simulink model "Finalproject342"  (R2014b)
settings: Solver=ode113  StartTime=0.0  StopTime=1200  RelTol=1e-3
undefined symbols (not defined in the file): ln
settings Model: Creator=mdbell  LastModifiedBy=Mike
settings DebuggingCC: MaxConsecutiveZCsMsg=none

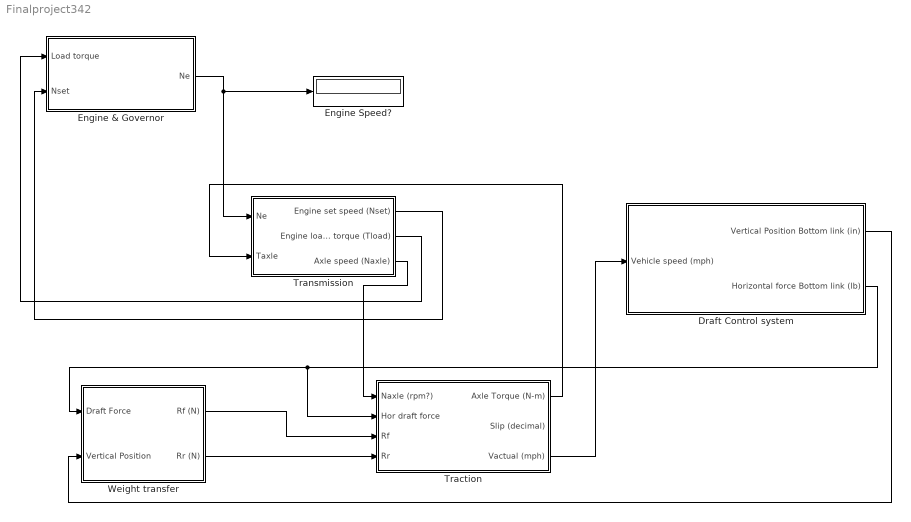
== system Finalproject342 ==
  Draft Control system : Subsystem
  Engine & Governor : Subsystem
  Engine Speed? : Display
  Traction : Subsystem
  Transmission : Subsystem
  Weight transfer : Subsystem
  wires:
  Engine & Governor/1(Ne) -> Transmission/1(Ne), Engine Speed?/1
  Transmission/1(Engine set speed (Nset)) -> Engine & Governor/2("Nset ")
  Draft Control system/2(Horizontal force Bottom link (lb)) -> Traction/2(Hor draft force), Weight transfer/1(Draft Force)
  Draft Control system/1(Vertical Position Bottom link (in)) -> Weight transfer/2(Vertical Position)
  Weight transfer/1(Rf (N)) -> Traction/3(Rf)
  Weight transfer/2(Rr (N)) -> Traction/4(Rr)
  Transmission/3(Axle speed (Naxle)) -> Traction/1(Naxle (rpm?))
  Traction/1(Axle Torque (N-m)) -> Transmission/2(Taxle)
  Traction/3(Vactual (mph)) -> Draft Control system/1(Vehicle speed (mph))
  Transmission/2(Engine load torque (Tload)) -> Engine & Governor/1(Load torque)

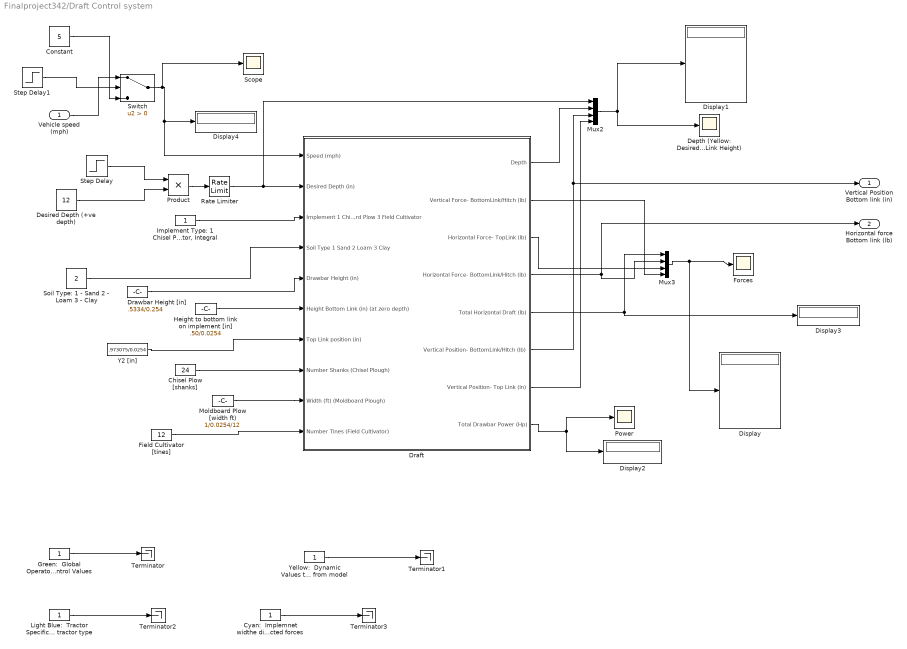
== system Finalproject342/Draft Control system ==
  Vehicle speed (mph) : Inport
  Chisel Plow [shanks] : Constant  Value=24
  Constant : Constant  Value=5
  Cyan:  Implemnet widthe dimension values to be changed to fit tractor type expected forces : Constant  OutDataTypeStr=int16
  "Depth (Yellow: Desired Depth, Purple: Actual Depth, Blue: Bottom Link Height, Red: Top Link Height) " : Scope
      settings: YMin=-0.5  YMax=1  SaveName=ScopeData27
  Desired Depth (+ve depth) : Constant  Value=12
  Display{,1..4} (5 alike) : Display
  "Draft " : Subsystem
  Drawbar Height [in] : Constant  Value=.5334/0.254
  Field Cultivator [tines] : Constant  Value=12
  Forces : Scope
      settings: YMin=-1000  YMax=4000  SaveName=ScopeData28
  Green:  Global Operator Control Values : Constant  OutDataTypeStr=int16
  Height to bottom link on implement [in] : Constant  Value=.50/0.0254
  "Implement Type: 1 Chisel Plough, Towed 2 Moldboard Plow, Semi Mounted 3 Field Cultivator, Integral" : Constant  OutDataTypeStr=int16
  Light Blue:  Tractor Specific dimension values to be changed to fit tractor type : Constant  OutDataTypeStr=int16
  Moldboard Plow [width ft) : Constant  Value=1/0.0254/12
  Mux2 : Mux
  Mux3 : Mux
  Power : Scope
      settings: YMin=0  YMax=400  SaveName=ScopeData29
  Product : Product  RndMeth=Zero
  Rate Limiter : RateLimiter  RisingSlewLimit=.1  FallingSlewLimit=-.1  SampleTimeMode=inherited
  Scope : Scope
      settings: TimeRange=2500  SaveName=ScopeData50
  Soil Type: 1 - Sand 2 - Loam 3 - Clay : Constant  Value=2
  Step Delay : Step  Time=500  SampleTime=0  ZeroCross=off
  Step Delay1 : Step  Time=50  After=500  SampleTime=0  ZeroCross=off
  Switch : Switch  Criteria=u2 > Threshold
  Terminator{,1..3} (4 alike) : Terminator
  "Y2 [in]   " : Constant  Value=.973075/0.0254
  Yellow:  Dynamic Values that need to be fed from model : Constant  OutDataTypeStr=int16
  Vertical Position Bottom link (in) : Outport
  Horizontal force Bottom link (lb) : Outport  Port=2
  wires:
  Mux3/1 -> Forces/1, Display/1
  "Draft "/7(Vertical Position- Top Link (in)) -> Mux2/4
  "Draft "/6(Vertical Position- BottomLink/Hitch (lb)) -> Vertical Position Bottom link (in)/1, Mux2/3
  "Draft "/5(Total Horizontal Draft (lb)) -> Display3/1, Mux3/1
  Moldboard Plow [width ft)/1 -> "Draft "/9(Width (ft) (Moldboard Plough))
  Field Cultivator [tines]/1 -> "Draft "/10(Number Tines (Field Cultivator))
  Desired Depth (+ve depth)/1 -> Product/2
  Green:  Global Operator Control Values/1 -> Terminator/1
  "Y2 [in]   "/1 -> "Draft "/7(Top Link position (in))
  "Implement Type: 1 Chisel Plough, Towed 2 Moldboard Plow, Semi Mounted 3 Field Cultivator, Integral"/1 -> "Draft "/3(Implement 1 Chisel Plough 2 Moldboard Plow 3 Field Cultivator)
  Drawbar Height [in]/1 -> "Draft "/5(Drawbar Height (in))
  "Draft "/4(Horizontal Force- BottomLink/Hitch (lb)) -> Mux3/2, Horizontal force Bottom link (lb)/1
  Chisel Plow [shanks]/1 -> "Draft "/8(Number Shanks (Chisel Plough))
  Yellow:  Dynamic Values that need to be fed from model/1 -> Terminator1/1
  Light Blue:  Tractor Specific dimension values to be changed to fit tractor type/1 -> Terminator2/1
  Cyan:  Implemnet widthe dimension values to be changed to fit tractor type expected forces/1 -> Terminator3/1
  "Draft "/8(Total Drawbar Power (Hp)) -> Power/1, Display2/1
  "Draft "/3(Horizontal Force- TopLink (lb)) -> Mux3/3
  Step Delay/1 -> Product/1
  Product/1 -> Rate Limiter/1
  Rate Limiter/1 -> "Draft "/2(Desired Depth (in)), Mux2/1
  Mux2/1 -> "Depth (Yellow: Desired Depth, Purple: Actual Depth, Blue: Bottom Link Height, Red: Top Link Height) "/1, Display1/1
  Soil Type: 1 - Sand 2 - Loam 3 - Clay/1 -> "Draft "/4(Soil Type 1 Sand 2 Loam 3 Clay)
  Height to bottom link on implement [in]/1 -> "Draft "/6(Height Bottom Link (in) (at zero depth))
  "Draft "/1(Depth) -> Mux2/2
  "Draft "/2(Vertical Force- BottomLink/Hitch (lb)) -> Mux3/4
  Step Delay1/1 -> Switch/2
  Switch/1 -> Scope/1, Display4/1, "Draft "/1(Speed (mph))
  Vehicle speed (mph)/1 -> Switch/1
  Constant/1 -> Switch/3

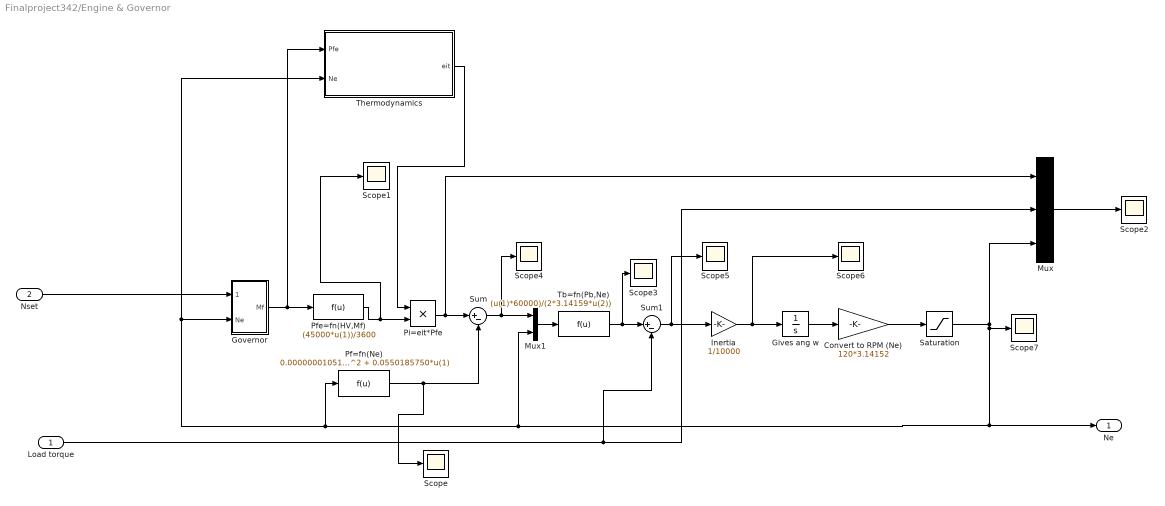
== system Finalproject342/Engine & Governor ==
  Load torque : Inport
  "Nset " : Inport  Port=2
  Convert to RPM (Ne) : Gain  Gain=120*3.14152
  Gives ang w : Integrator  UpperSaturationLimit=1  LowerSaturationLimit=0
  Governor : Subsystem
  Inertia : Gain  Gain=1/10000
  Mux : Mux  Inputs=3
  Mux1 : Mux  Inputs=2
  Pf=fn(Ne) : Fcn  Expr=0.00000001051*u(1)^3 - 0.00003889215*u(1)^2 + 0.0550185750*u(1)
  Pfe=fn(HV,Mf) : Fcn  Expr=(45000*u(1))/3600
  Pi=eit*Pfe : Product
  Saturation : Saturate  UpperLimit=5000  LowerLimit=1000
  Scope{,1..7} (8 alike) : Scope
      Scope2 settings: SaveName=ScopeData15
      Scope3 settings: SaveName=ScopeData6
      Scope4 settings: SaveName=ScopeData7
      Scope5 settings: SaveName=ScopeData8
      Scope6 settings: SaveName=ScopeData10
      Scope7 settings: SaveName=ScopeData11
  Sum : Sum  Inputs=|+-
  Sum1 : Sum  Inputs=|+-
  Tb=fn(Pb,Ne) : Fcn  Expr=(u(1)*60000)/(2*3.14159*u(2))
  Thermodynamics : Subsystem
  Ne : Outport
  wires:
  Load torque/1 -> Mux/2, Sum1/2
  "Nset "/1 -> Governor/1(NeSet)
  Pfe=fn(HV,Mf)/1 -> Scope1/1, Pi=eit*Pfe/2
  Pi=eit*Pfe/1 -> Mux/1, Sum/1
  Pf=fn(Ne)/1 -> Scope/1, Sum/2
  Sum/1 -> Scope4/1, Mux1/1
  Mux1/1 -> Tb=fn(Pb,Ne)/1
  Tb=fn(Pb,Ne)/1 -> Scope3/1, Sum1/1
  Sum1/1 -> Scope5/1, Inertia/1
  Inertia/1 -> Scope6/1, Gives ang w/1
  Gives ang w/1 -> Convert to RPM (Ne)/1
  Convert to RPM (Ne)/1 -> Saturation/1
  Mux/1 -> Scope2/1
  Saturation/1 -> Mux/3, Mux1/2, Pf=fn(Ne)/1, Thermodynamics/2(Ne), Governor/2(Ne), Ne/1, Scope7/1
  Governor/1(Mf) -> Thermodynamics/1(Pfe), Pfe=fn(HV,Mf)/1
  Thermodynamics/1("eit ") -> Pi=eit*Pfe/1

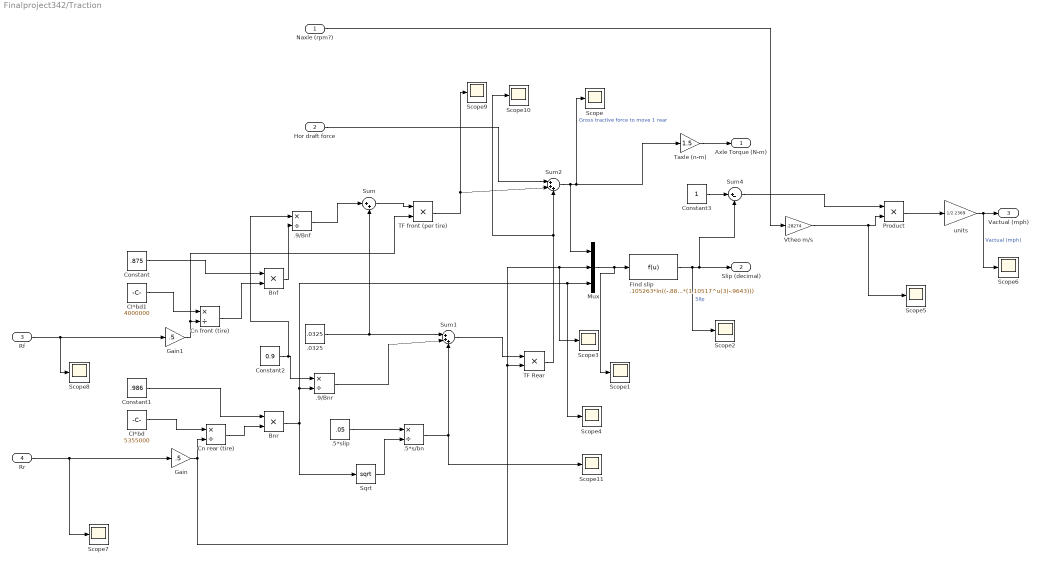
== system Finalproject342/Traction ==
  Naxle (rpm?) : Inport
  Hor draft force : Inport  Port=2
  Rf : Inport  Port=3
  Rr : Inport  Port=4
  .0325 : Constant  Value=.0325
  .5*s/bn : Product  Inputs=*/
  .5*slip : Constant  Value=.05
  .9/Bnf : Product  Inputs=*/
  .9/Bnr : Product  Inputs=*/
  Bnf : Product
  Bnr : Product
  CI*bd : Constant  Value=5355000
  CI*bd1 : Constant  Value=4000000
  Cn front (tire) : Product  Inputs=*/
  Cn rear (tire) : Product  Inputs=*/
  Constant : Constant  Value=.875
  Constant1 : Constant  Value=.986
  Constant2 : Constant  Value=0.9
  Constant3 : Constant
  Find slip : Fcn  Expr=.105263*ln((-.88*(1.10517^u(3)-1))/((u(1)/u(2))*1.10517^u(3)-.9125*(1.10517^u(3)-.9643)))
  Gain : Gain  Gain=.5
  Gain1 : Gain  Gain=.5
  Mux : Mux  Inputs=3
  Product : Product
  Scope{,1..11} (12 alike) : Scope
      Scope settings: SaveName=ScopeData30
      Scope1 settings: SaveName=ScopeData31
      Scope10 settings: SaveName=ScopeData46
      Scope11 settings: SaveName=ScopeData47
      Scope2 settings: ShowLegends=on  SaveName=ScopeData32
      Scope3 settings: SaveName=ScopeData33
      Scope4 settings: SaveName=ScopeData34
      Scope5 settings: SaveName=ScopeData35
      Scope6 settings: ShowLegends=on  YMin=-0  YMax=10  SaveName=ScopeData36
      Scope7 settings: SaveName=ScopeData37
      Scope8 settings: SaveName=ScopeData38
      Scope9 settings: SaveName=ScopeData45
  Sqrt : Sqrt  OutputSignalType=real  SaturateOnIntegerOverflow=on
  Sum : Sum  Inputs=|++
  Sum1 : Sum  Inputs=|+++
  Sum2 : Sum  Inputs=|+++
  Sum4 : Sum  Inputs=|+-
  TF Rear : Product
  TF front (per tire) : Product
  Taxle (n-m) : Gain  Gain=1.5
  Vtheo m/s : Gain  Gain=.28274
  units : Gain  Gain=1/2.2369
  Axle Torque (N-m) : Outport
  Slip (decimal) : Outport  Port=2
  Vactual (mph) : Outport  Port=3
  wires:
  CI*bd/1 -> Cn rear (tire)/1
  Rr/1 -> Scope7/1, Gain/1
  Gain/1 -> Mux/2, Scope3/1, TF Rear/2, Cn rear (tire)/2
  CI*bd1/1 -> Cn front (tire)/1
  Rf/1 -> Scope8/1, Gain1/1
  Gain1/1 -> TF front (per tire)/2, Cn front (tire)/2
  Cn front (tire)/1 -> Bnf/2
  Constant/1 -> Bnf/1
  Constant1/1 -> Bnr/1
  Cn rear (tire)/1 -> Bnr/2
  Constant2/1 -> .9/Bnf/1, .9/Bnr/1
  .0325/1 -> Sum1/1, Sum/2
  .9/Bnr/1 -> Sum1/2
  .9/Bnf/1 -> Sum/1
  Sum/1 -> TF front (per tire)/1
  .5*slip/1 -> .5*s/bn/1
  .5*s/bn/1 -> Sum1/3, Scope11/1
  Sum1/1 -> TF Rear/1
  TF Rear/1 -> Scope10/1, Sum2/3
  TF front (per tire)/1 -> Scope9/1, Sum2/2
  Hor draft force/1 -> Sum2/1
  Sum2/1 -> Mux/1, Scope/1, Taxle (n-m)/1  "Gross tractive force to move 1 rear"
  Taxle (n-m)/1 -> Axle Torque (N-m)/1
  Sqrt/1 -> .5*s/bn/2
  Bnf/1 -> .9/Bnf/2
  Mux/1 -> Scope1/1, Find slip/1
  Find slip/1 -> Scope2/1, Sum4/2, Slip (decimal)/1  "Slip"
  Naxle (rpm?)/1 -> Vtheo m/s/1
  Constant3/1 -> Sum4/1
  Sum4/1 -> Product/1
  Product/1 -> units/1
  Bnr/1 -> Sqrt/1, Scope4/1, Mux/3, .9/Bnr/2
  units/1 -> Vactual (mph)/1, Scope6/1  "Vactual (mph)"
  Vtheo m/s/1 -> Scope5/1, Product/2

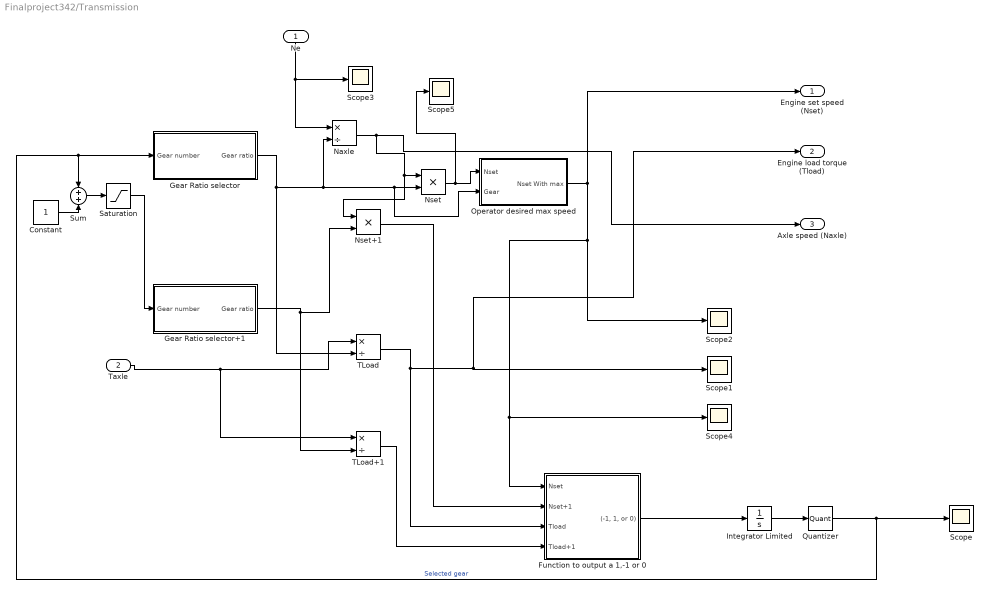
== system Finalproject342/Transmission ==
  Ne : Inport
  Taxle : Inport  Port=2
  Constant : Constant
  Function to output a 1,-1 or 0 : Subsystem
  Gear Ratio selector : Subsystem
  Gear Ratio selector+1 : Subsystem
  Integrator Limited : Integrator  InitialCondition=5  LimitOutput=on  UpperSaturationLimit=16  LowerSaturationLimit=1
  Naxle : Product  Inputs=*/
  Nset : Product
  Nset+1 : Product
  Operator desired max speed : Subsystem
  Quantizer : Quantizer  QuantizationInterval=1
  Saturation : Saturate  UpperLimit=16  LowerLimit=0  ZeroCross=off
  Scope{,1..5} (6 alike) : Scope
      Scope settings: ShowLegends=on  SaveName=ScopeData54
      Scope1 settings: SaveName=ScopeData21
      Scope2 settings: SaveName=ScopeData26
      Scope3 settings: ShowLegends=on  SaveName=ScopeData20
      Scope4 settings: SaveName=ScopeData48
      Scope5 settings: SaveName=ScopeData44
  Sum : Sum  Inputs=+|+
  TLoad : Product  Inputs=*/
  TLoad+1 : Product  Inputs=*/
  Engine set speed (Nset) : Outport
  Engine load torque (Tload) : Outport  Port=2
  Axle speed (Naxle) : Outport  Port=3
  wires:
  Function to output a 1,-1 or 0/1("(-1, 1, or 0)") -> Integrator Limited/1
  Quantizer/1 -> Scope/1, Sum/1, Gear Ratio selector/1(Gear number)  "Selected gear"
  Nset+1/1 -> Function to output a 1,-1 or 0/2(Nset+1)
  Gear Ratio selector+1/1(Gear ratio) -> TLoad+1/2, Nset+1/2
  TLoad+1/1 -> Function to output a 1,-1 or 0/4(Tload+1)
  Constant/1 -> Sum/2
  Gear Ratio selector/1(Gear ratio) -> TLoad/2, Naxle/2, Operator desired max speed/2(Gear), Nset/2
  Taxle/1 -> TLoad+1/1, TLoad/1
  TLoad/1 -> Function to output a 1,-1 or 0/3(Tload), Engine load torque (Tload)/1, Scope1/1
  Saturation/1 -> Gear Ratio selector+1/1(Gear number)
  Sum/1 -> Saturation/1
  Integrator Limited/1 -> Quantizer/1
  Ne/1 -> Naxle/1, Scope3/1
  Operator desired max speed/1(Nset With max) -> Engine set speed (Nset)/1, Function to output a 1,-1 or 0/1(Nset), Scope4/1, Scope2/1
  Nset/1 -> Scope5/1, Operator desired max speed/1(Nset)
  Naxle/1 -> Nset+1/1, Nset/1, Axle speed (Naxle)/1

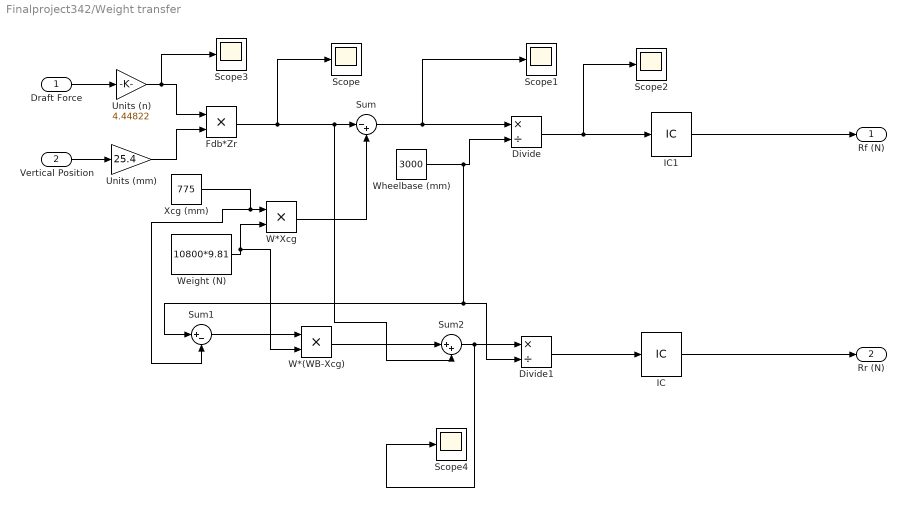
== system Finalproject342/Weight transfer ==
  Draft Force : Inport
  Vertical Position : Inport  Port=2
  Divide : Product  Inputs=*/
  Divide1 : Product  Inputs=*/
  Fdb*Zr : Product
  IC : InitialCondition  Value=70
  IC1 : InitialCondition  Value=50
  Scope{,1..4} (5 alike) : Scope
      Scope settings: SaveName=ScopeData39
      Scope1 settings: SaveName=ScopeData40
      Scope2 settings: SaveName=ScopeData41
      Scope3 settings: SaveName=ScopeData42
      Scope4 settings: SaveName=ScopeData43
  Sum : Sum  Inputs=|-+
  Sum1 : Sum  Inputs=|+-
  Sum2 : Sum  Inputs=|++
  Units (mm) : Gain  Gain=25.4
  Units (n) : Gain  Gain=4.44822
  W*(WB-Xcg) : Product
  W*Xcg : Product
  Weight (N) : Constant  Value=10800*9.81
  Wheelbase (mm) : Constant  Value=3000
  Xcg (mm) : Constant  Value=775
  Rf (N) : Outport
  Rr (N) : Outport  Port=2
  wires:
  Xcg (mm)/1 -> Sum1/2, W*Xcg/1
  Weight (N)/1 -> W*(WB-Xcg)/2, W*Xcg/2
  Draft Force/1 -> Units (n)/1
  Units (n)/1 -> Scope3/1, Fdb*Zr/1
  Vertical Position/1 -> Units (mm)/1
  Units (mm)/1 -> Fdb*Zr/2
  Fdb*Zr/1 -> Scope/1, Sum/1, Sum2/2
  W*Xcg/1 -> Sum/2
  Sum/1 -> Scope1/1, Divide/1
  Wheelbase (mm)/1 -> Divide1/2, Sum1/1, Divide/2
  Divide/1 -> Scope2/1, IC1/1
  Sum1/1 -> W*(WB-Xcg)/1
  W*(WB-Xcg)/1 -> Sum2/1
  Sum2/1 -> Scope4/1, Divide1/1
  Divide1/1 -> IC/1
  IC/1 -> Rr (N)/1
  IC1/1 -> Rf (N)/1

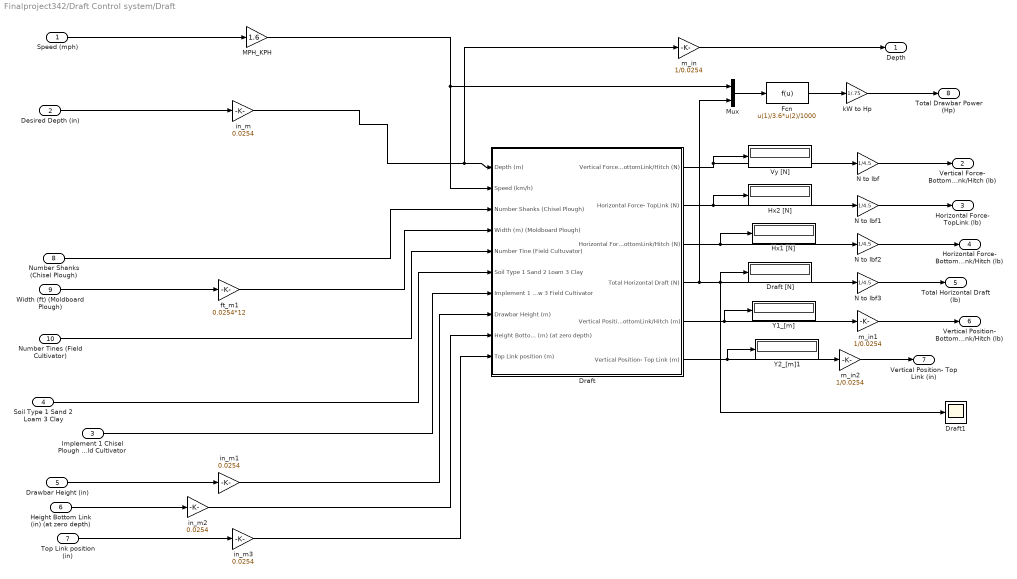
== system Finalproject342/Draft Control system/Draft  ==
  Speed (mph) : Inport  OutDataTypeStr=double
  Desired Depth (in) : Inport  Port=2
  Implement 1 Chisel Plough 2 Moldboard Plow 3 Field Cultivator : Inport  Port=3
  Soil Type 1 Sand 2 Loam 3 Clay : Inport  Port=4
  Drawbar Height (in) : Inport  Port=5
  Height Bottom Link (in) (at zero depth) : Inport  Port=6
  Top Link position (in) : Inport  Port=7
  Number Shanks (Chisel Plough) : Inport  Port=8
  Width (ft) (Moldboard Plough) : Inport  Port=9
  Number Tines (Field Cultivator) : Inport  Port=10
  Draft : Subsystem
  Draft [N] : Display
      settings: Format=bank
  Draft1 : Scope
      settings: YMin=0  YMax=1e+006  SaveName=ScopeData3
  Fcn : Fcn  Expr=u(1)/3.6*u(2)/1000
  "Hx1 [N] " : Display
      settings: Format=bank
  Hx2 [N] : Display
      settings: Format=bank
  MPH_KPH : Gain  Gain=1.6
  Mux : Mux  Inputs=2
  N to lbf{,1..3} (4 alike) : Gain  Gain=1/4.5
  Vy [N] : Display
      settings: Format=bank
  Y1_[m] : Display
      settings: Format=bank
  Y2_[m]1 : Display
      settings: Format=bank
  ft_m1 : Gain  Gain=0.0254*12
  in_m{,1..3} (4 alike) : Gain  Gain=0.0254
  kW to Hp : Gain  Gain=1/.75
  m_in : Gain  Gain=1/0.0254
  m_in1 : Gain  Gain=1/0.0254
  m_in2 : Gain  Gain=1/0.0254
  Depth : Outport
  Vertical Force- BottomLink/Hitch (lb) : Outport  Port=2
  Horizontal Force- TopLink (lb) : Outport  Port=3
  Horizontal Force- BottomLink/Hitch (lb) : Outport  Port=4
  Total Horizontal Draft (lb) : Outport  Port=5
  Vertical Position- BottomLink/Hitch (lb) : Outport  Port=6
  Vertical Position- Top Link (in) : Outport  Port=7
  Total Drawbar Power (Hp) : Outport  Port=8
  wires:
  Draft/6(Vertical Position- Top Link (m)) -> Y2_[m]1/1, m_in2/1
  Draft/5(Vertical Position- BottomLink/Hitch (m)) -> Y1_[m]/1, m_in1/1
  Draft/1(Vertical Force- BottomLink/Hitch (N)) -> Vy [N]/1, N to lbf/1
  Draft/2(Horizontal Force- TopLink (N)) -> Hx2 [N]/1, N to lbf1/1
  Draft/3(Horizontal Force- BottomLink/Hitch (N)) -> "Hx1 [N] "/1, N to lbf2/1
  Draft/4(Total Horizontal Draft (N)) -> Draft [N]/1, Draft1/1, N to lbf3/1, Mux/2
  Desired Depth (in)/1 -> in_m/1
  Speed (mph)/1 -> MPH_KPH/1
  Soil Type 1 Sand 2 Loam 3 Clay/1 -> Draft/6(Soil Type 1 Sand 2 Loam 3 Clay)
  Drawbar Height (in)/1 -> in_m1/1
  Height Bottom Link (in) (at zero depth)/1 -> in_m2/1
  Top Link position (in)/1 -> in_m3/1
  Number Shanks (Chisel Plough)/1 -> Draft/3(Number Shanks (Chisel Plough))
  Width (ft) (Moldboard Plough)/1 -> ft_m1/1
  Number Tines (Field Cultivator)/1 -> Draft/5(Number Tine (Field Cultuvator))
  Implement 1 Chisel Plough 2 Moldboard Plow 3 Field Cultivator/1 -> Draft/7(Implement 1 Chisel Plough 2 Moldboard Plow 3 Field Cultivator)
  Mux/1 -> Fcn/1
  Fcn/1 -> kW to Hp/1
  MPH_KPH/1 -> Draft/2(Speed (km/h)), Mux/1
  in_m/1 -> Draft/1(Depth (m)), m_in/1
  ft_m1/1 -> Draft/4(Width (m) (Moldboard Plough))
  in_m1/1 -> Draft/8(Drawbar Height (m))
  in_m2/1 -> Draft/9(Height Bottom Link (m) (at zero depth))
  in_m3/1 -> Draft/10(Top Link position (m))
  m_in/1 -> Depth/1
  kW to Hp/1 -> Total Drawbar Power (Hp)/1
  m_in1/1 -> Vertical Position- BottomLink/Hitch (lb)/1
  m_in2/1 -> Vertical Position- Top Link (in)/1
  N to lbf/1 -> Vertical Force- BottomLink/Hitch (lb)/1
  N to lbf1/1 -> Horizontal Force- TopLink (lb)/1
  N to lbf2/1 -> Horizontal Force- BottomLink/Hitch (lb)/1
  N to lbf3/1 -> Total Horizontal Draft (lb)/1

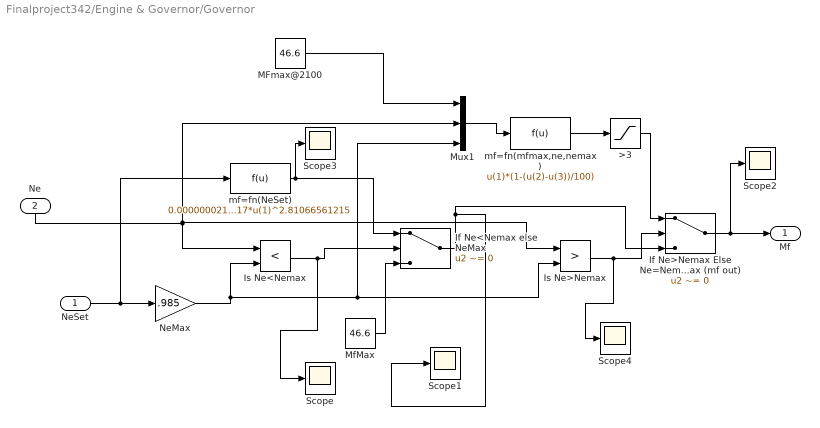
== system Finalproject342/Engine & Governor/Governor ==
  NeSet : Inport
  Ne : Inport  Port=2
  >3 : Saturate  UpperLimit=100  LowerLimit=3
  If Ne<Nemax else NeMax : Switch  Criteria=u2 ~= 0  Threshold=2068.5
  If Ne>Nemax Else Ne=Nemax (mf out) : Switch  Criteria=u2 ~= 0  Threshold=2068.5
  Is Ne<Nemax : RelationalOperator  Operator=<  OutDataTypeStr=boolean
  Is Ne>Nemax : RelationalOperator  Operator=>  OutDataTypeStr=boolean
  MFmax@2100 : Constant  Value=46.6
  MfMax : Constant  Value=46.6
  Mux1 : Mux  Inputs=3
  NeMax : Gain  Gain=.985
  Scope{,1..4} (5 alike) : Scope
      Scope settings: SaveName=ScopeData2
      Scope1 settings: SaveName=ScopeData3
      Scope2 settings: SaveName=ScopeData4
      Scope3 settings: SaveName=ScopeData9
      Scope4 settings: SaveName=ScopeData12
  mf=fn(NeSet) : Fcn  Expr=0.00000002117*u(1)^2.81066561215
  mf=fn(mfmax,ne,nemax) : Fcn  Expr=u(1)*(1-(u(2)-u(3))/100)
  Mf : Outport
  wires:
  mf=fn(NeSet)/1 -> Scope3/1, If Ne<Nemax else NeMax/1
  If Ne>Nemax Else Ne=Nemax (mf out)/1 -> Scope2/1, Mf/1
  MFmax@2100/1 -> Mux1/1
  NeSet/1 -> mf=fn(NeSet)/1, NeMax/1
  If Ne<Nemax else NeMax/1 -> Scope1/1, If Ne>Nemax Else Ne=Nemax (mf out)/3
  NeMax/1 -> Is Ne<Nemax/2, Is Ne>Nemax/2, Mux1/3
  Is Ne<Nemax/1 -> Scope/1, If Ne<Nemax else NeMax/2
  >3/1 -> If Ne>Nemax Else Ne=Nemax (mf out)/1
  mf=fn(mfmax,ne,nemax)/1 -> >3/1
  Mux1/1 -> mf=fn(mfmax,ne,nemax)/1
  Ne/1 -> Mux1/2, Is Ne>Nemax/1, Is Ne<Nemax/1
  Is Ne>Nemax/1 -> Scope4/1, If Ne>Nemax Else Ne=Nemax (mf out)/2
  MfMax/1 -> If Ne<Nemax else NeMax/3

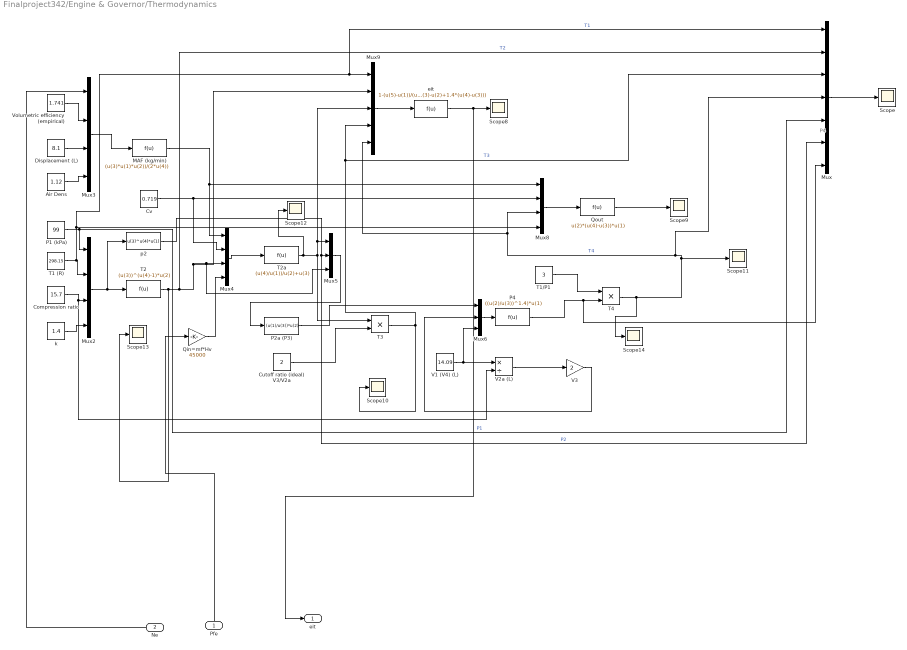
== system Finalproject342/Engine & Governor/Thermodynamics ==
  note: P4
  Pfe : Inport
  Ne : Inport  Port=2
  Air Dens : Constant  Value=1.12
  Compression ratio : Constant  Value=15.7
  Cutoff ratio (ideal) V3/V2a : Constant  Value=2
  Cv : Constant  Value=0.719
  Displacement (L) : Constant  Value=8.1
  MAF (kg/min) : Fcn  Expr=(u(3)*u(1)*u(2))/(2*u(4))
  Mux : Mux  Inputs=7
  Mux{2..4,8} (4 alike) : Mux
  Mux5 : Mux  Inputs=3
  Mux6 : Mux  Inputs=3
  Mux9 : Mux  Inputs=5
  P1 (kPa) : Constant  Value=99
  P2a (P3) : Fcn  Expr=(u(1)/u(3))*u(2)
  P4 : Fcn  Expr=((u(2)/u(3))^1.4)*u(1)
  Qin=mf*Hv : Gain  Gain=45000
  Qout : Fcn  Expr=u(2)*(u(4)-u(3))*u(1)
  Scope{,8..14} (8 alike) : Scope
      Scope settings: ShowLegends=on  SaveName=ScopeData52
      Scope10 settings: SaveName=ScopeData14
      Scope11 settings: SaveName=ScopeData16
      Scope12 settings: SaveName=ScopeData17
      Scope13 settings: SaveName=ScopeData18
      Scope14 settings: SaveName=ScopeData19
      Scope8 settings: ShowLegends=on  TimeRange=104.5627376425857  YMin=0.617825  YMax=0.618375  SaveName=ScopeData5
      Scope9 settings: SaveName=ScopeData13
  T1 (R) : Constant  Value=298.15
  T1/P1 : Constant  Value=3
  T2 : Fcn  Expr=(u(3))^(u(4)-1)*u(2)
  T2a : Fcn  Expr=(u(4)/u(1))/u(2)+u(3)
  T3 : Product
  T4 : Product
  V1 (V4) (L) : Constant  Value=14.09
  V2a (L) : Product  Inputs=*/
  V3 : Gain  Gain=2
  Volumetric efficiency (empirical) : Constant  Value=1.741
  eit : Fcn  Expr=1-(u(5)-u(1))/(u(3)-u(2)+1.4*(u(4)-u(3)))
  k : Constant  Value=1.4
  p2 : Fcn  Expr=u(3)^u(4)*u(1)
  "eit " : Outport
  wires:
  Volumetric efficiency (empirical)/1 -> Mux3/2
  Displacement (L)/1 -> Mux3/3
  Mux2/1 -> T2/1, p2/1
  k/1 -> Mux2/4
  eit/1 -> "eit "/1, Scope8/1
  Air Dens/1 -> Mux3/4
  Mux3/1 -> MAF (kg/min)/1
  T2a/1 -> Scope12/1, T3/1, Mux9/3, Mux5/1
  Compression ratio/1 -> V2a (L)/2, Mux2/3
  Cv/1 -> Mux8/2, Mux4/2
  Mux5/1 -> P2a (P3)/1
  Mux8/1 -> Qout/1
  Mux6/1 -> P4/1
  T3/1 -> Scope10/1, Mux/3, Mux9/4  "T3"
  MAF (kg/min)/1 -> Mux8/1, Mux4/1
  T4/1 -> Scope14/1, Scope11/1, Mux/4, Mux8/3, Mux9/5  "T4"
  T2/1 -> Scope13/1, Mux/2, Mux9/2, Mux5/3, Mux4/3  "T2"
  Qout/1 -> Scope9/1
  p2/1 -> Mux/6, Mux5/2  "P2"
  Cutoff ratio (ideal) V3/V2a/1 -> T3/2
  Qin=mf*Hv/1 -> Mux4/4
  T1 (R)/1 -> Mux/1, Mux9/1, Mux8/4, Mux2/2  "T1"
  P4/1 -> Mux/7, T4/2
  Mux9/1 -> eit/1
  P1 (kPa)/1 -> Mux2/1, Mux/5  "P1"
  T1/P1/1 -> T4/1
  V1 (V4) (L)/1 -> Mux6/3, V2a (L)/1
  Mux4/1 -> T2a/1
  V2a (L)/1 -> V3/1
  V3/1 -> Mux6/2
  P2a (P3)/1 -> Mux6/1
  Ne/1 -> Mux3/1
  Pfe/1 -> Qin=mf*Hv/1
  Mux/1 -> Scope/1

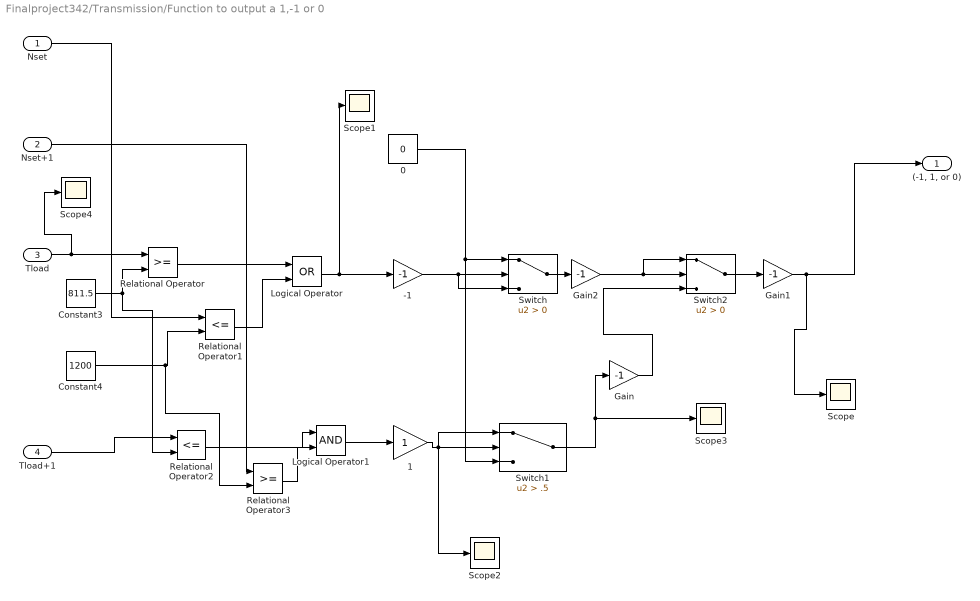
== system Finalproject342/Transmission/Function to output a 1,-1 or 0 ==
  Nset : Inport
  Nset+1 : Inport  Port=2
  Tload : Inport  Port=3
  Tload+1 : Inport  Port=4
  -1 : Gain  Gain=-1
  0 : Constant  Value=0
  1 : Gain
  Constant3 : Constant  Value=811.5
  Constant4 : Constant  Value=1200
  Gain : Gain  Gain=-1
  Gain1 : Gain  Gain=-1
  Gain2 : Gain  Gain=-1
  Logical Operator : Logic  Operator=OR  AllPortsSameDT=off  OutDataTypeStr=boolean
  Logical Operator1 : Logic  AllPortsSameDT=off  OutDataTypeStr=boolean
  Relational Operator : RelationalOperator  OutDataTypeStr=boolean  ZeroCross=off
  Relational Operator1 : RelationalOperator  Operator=<=  OutDataTypeStr=boolean  ZeroCross=off
  Relational Operator2 : RelationalOperator  Operator=<=  OutDataTypeStr=boolean  ZeroCross=off
  Relational Operator3 : RelationalOperator  OutDataTypeStr=boolean  ZeroCross=off
  Scope{,1..4} (5 alike) : Scope
      Scope settings: SaveName=ScopeData22
      Scope1 settings: SaveName=ScopeData23
      Scope2 settings: SaveName=ScopeData24
      Scope3 settings: SaveName=ScopeData25
      Scope4 settings: SaveName=ScopeData49
  Switch : Switch  Criteria=u2 > Threshold  ZeroCross=off
  Switch1 : Switch  Criteria=u2 > Threshold  Threshold=.5  ZeroCross=off
  Switch2 : Switch  Criteria=u2 > Threshold  ZeroCross=off
  "(-1, 1, or 0)" : Outport
  wires:
  Tload/1 -> Scope4/1, Relational Operator/1
  Constant3/1 -> Relational Operator/2, Relational Operator2/2
  Relational Operator/1 -> Logical Operator/1
  Nset/1 -> Relational Operator1/1
  Constant4/1 -> Relational Operator3/2, Relational Operator1/2
  Relational Operator1/1 -> Logical Operator/2
  Logical Operator/1 -> Scope1/1, -1/1
  Tload+1/1 -> Relational Operator2/1
  Relational Operator2/1 -> Logical Operator1/1
  Relational Operator3/1 -> Logical Operator1/2
  Logical Operator1/1 -> 1/1
  -1/1 -> Switch/3, Switch/2
  0/1 -> Switch1/3, Switch/1
  1/1 -> Switch1/2, Scope2/1, Switch1/1
  Switch/1 -> Gain2/1
  Switch1/1 -> Scope3/1, Gain/1
  Gain/1 -> Switch2/3
  Switch2/1 -> Gain1/1
  Nset+1/1 -> Relational Operator3/1
  Gain1/1 -> "(-1, 1, or 0)"/1, Scope/1
  Gain2/1 -> Switch2/1, Switch2/2

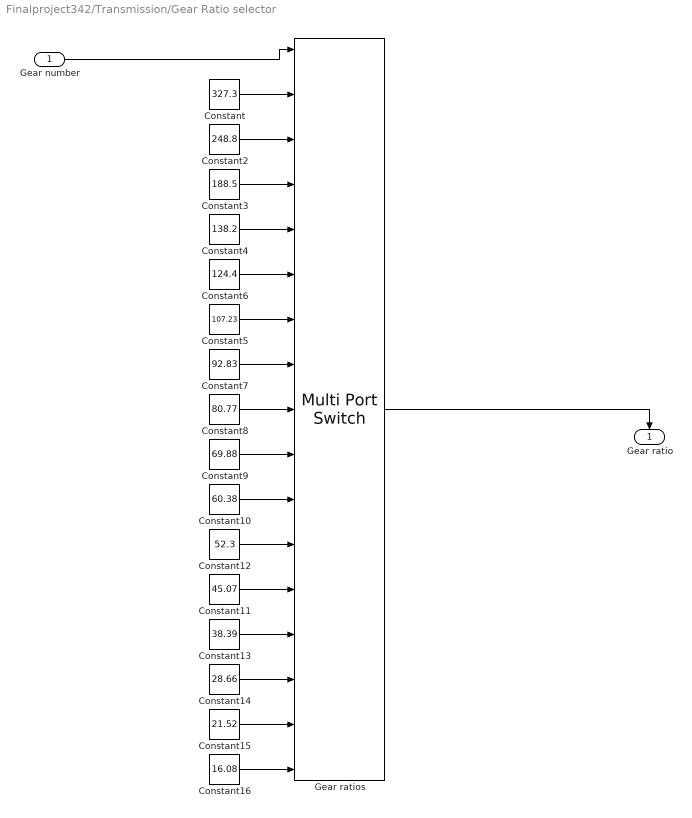
== system Finalproject342/Transmission/Gear Ratio selector ==
  Gear number : Inport
  Constant : Constant  Value=327.3
  Constant10 : Constant  Value=60.38
  Constant11 : Constant  Value=45.07
  Constant12 : Constant  Value=52.3
  Constant13 : Constant  Value=38.39
  Constant14 : Constant  Value=28.66
  Constant15 : Constant  Value=21.52
  Constant16 : Constant  Value=16.08
  Constant2 : Constant  Value=248.8
  Constant3 : Constant  Value=188.5
  Constant4 : Constant  Value=138.2
  Constant5 : Constant  Value=107.23
  Constant6 : Constant  Value=124.4
  Constant7 : Constant  Value=92.83
  Constant8 : Constant  Value=80.77
  Constant9 : Constant  Value=69.88
  Gear ratios : MultiPortSwitch  Inputs=16
  Gear ratio : Outport
  wires:
  Constant4/1 -> Gear ratios/5
  Constant9/1 -> Gear ratios/10
  Constant14/1 -> Gear ratios/15
  Constant15/1 -> Gear ratios/16
  Gear number/1 -> Gear ratios/1
  Constant8/1 -> Gear ratios/9
  Constant13/1 -> Gear ratios/14
  Constant11/1 -> Gear ratios/13
  Constant5/1 -> Gear ratios/7
  Constant/1 -> Gear ratios/2
  Constant2/1 -> Gear ratios/3
  Constant7/1 -> Gear ratios/8
  Constant10/1 -> Gear ratios/11
  Constant3/1 -> Gear ratios/4
  Gear ratios/1 -> Gear ratio/1
  Constant6/1 -> Gear ratios/6
  Constant12/1 -> Gear ratios/12
  Constant16/1 -> Gear ratios/17

== system Finalproject342/Transmission/Gear Ratio selector+1 ==
  Gear number : Inport
  Constant : Constant  Value=327.3
  Constant10 : Constant  Value=60.38
  Constant11 : Constant  Value=45.07
  Constant12 : Constant  Value=52.3
  Constant13 : Constant  Value=38.39
  Constant14 : Constant  Value=28.66
  Constant15 : Constant  Value=21.52
  Constant16 : Constant  Value=16.08
  Constant2 : Constant  Value=248.8
  Constant3 : Constant  Value=188.5
  Constant4 : Constant  Value=138.2
  Constant5 : Constant  Value=107.23
  Constant6 : Constant  Value=124.4
  Constant7 : Constant  Value=92.83
  Constant8 : Constant  Value=80.77
  Constant9 : Constant  Value=69.88
  Gear ratios : MultiPortSwitch  Inputs=16
  Gear ratio : Outport
  wires:
  Constant4/1 -> Gear ratios/5
  Constant9/1 -> Gear ratios/10
  Constant14/1 -> Gear ratios/15
  Constant15/1 -> Gear ratios/16
  Gear number/1 -> Gear ratios/1
  Constant8/1 -> Gear ratios/9
  Constant13/1 -> Gear ratios/14
  Constant11/1 -> Gear ratios/13
  Constant5/1 -> Gear ratios/7
  Constant/1 -> Gear ratios/2
  Constant2/1 -> Gear ratios/3
  Constant7/1 -> Gear ratios/8
  Constant10/1 -> Gear ratios/11
  Constant3/1 -> Gear ratios/4
  Gear ratios/1 -> Gear ratio/1
  Constant6/1 -> Gear ratios/6
  Constant12/1 -> Gear ratios/12
  Constant16/1 -> Gear ratios/17

== system Finalproject342/Transmission/Operator desired max speed ==
  Nset : Inport
  Gear : Inport  Port=2
  Desired speed km/h : Constant  Value=50
  Naxle set : Product  Inputs=*/
  Product : Product
  Rate Limiter : RateLimiter  RisingSlewLimit=2  FallingSlewLimit=-2  SampleTimeMode=inherited
  Relational Operator : RelationalOperator  Operator=>  OutDataTypeStr=boolean
  Saturation : Saturate  UpperLimit=2400  LowerLimit=0
  Scope : Scope
      settings: TimeRange=482.4482481598204  YMin=26.12499999999999  YMax=34.37499999999999  SaveName=ScopeData51
  Switch : Switch  Criteria=u2 > Threshold
  Vtheo m/s : Gain  Gain=.28274
  Vtheo m/s1 : Gain  Gain=1/.28274
  Nset With max : Outport
  wires:
  Nset/1 -> Naxle set/1
  Gear/1 -> Product/2, Naxle set/2
  Naxle set/1 -> Vtheo m/s/1
  Vtheo m/s/1 -> Switch/3, Relational Operator/2
  Relational Operator/1 -> Switch/2
  Switch/1 -> Scope/1, Vtheo m/s1/1
  Vtheo m/s1/1 -> Product/1
  Product/1 -> Saturation/1
  Saturation/1 -> Rate Limiter/1
  Rate Limiter/1 -> Nset With max/1
  Desired speed km/h/1 -> Switch/1, Relational Operator/1

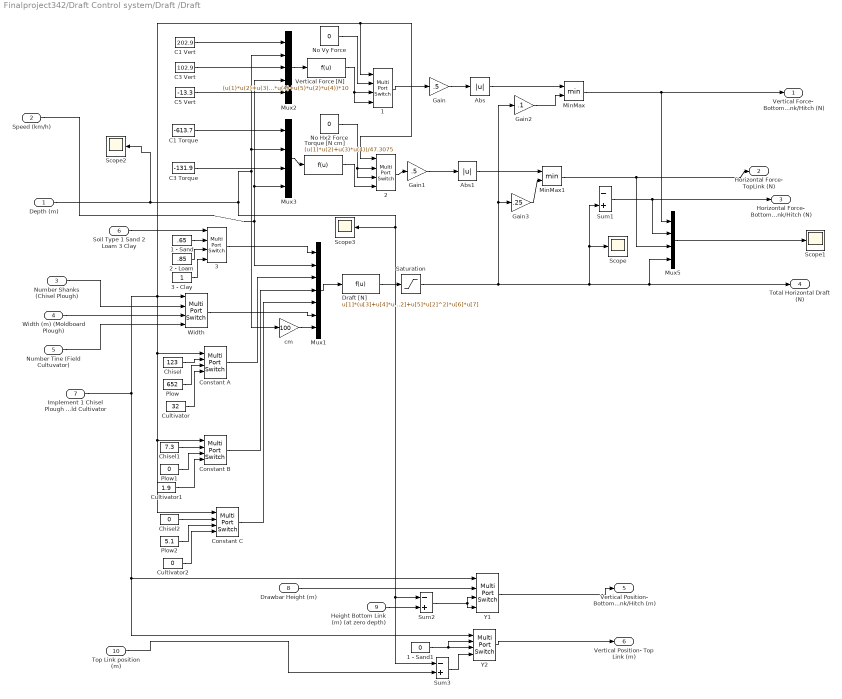
== system Finalproject342/Draft Control system/Draft /Draft ==
  Depth (m) : Inport
  Speed (km/h) : Inport  Port=2
  Number Shanks (Chisel Plough) : Inport  Port=3
  Width (m) (Moldboard Plough) : Inport  Port=4
  Number Tine (Field Cultuvator) : Inport  Port=5
  Soil Type 1 Sand 2 Loam 3 Clay : Inport  Port=6
  Implement 1 Chisel Plough 2 Moldboard Plow 3 Field Cultivator : Inport  Port=7
  Drawbar Height (m) : Inport  Port=8
  Height Bottom Link (m) (at zero depth) : Inport  Port=9
  Top Link position (m) : Inport  Port=10
  1 : MultiPortSwitch  SaturateOnIntegerOverflow=on  InputSameDT=on
  1 - Sand : Constant  Value=.65
  1 - Sand1 : Constant  Value=0
  2 : MultiPortSwitch  SaturateOnIntegerOverflow=on  InputSameDT=on
  2 - Loam : Constant  Value=.85
  3 : MultiPortSwitch  SaturateOnIntegerOverflow=on  InputSameDT=on
  3 - Clay : Constant
  Abs : Abs
  Abs1 : Abs
  C1 Torque : Constant  Value=-613.7
  C1 Vert : Constant  Value=202.9
  C3 Torque : Constant  Value=-131.9
  C3 Vert : Constant  Value=102.9
  C5 Vert : Constant  Value=-13.3
  Chisel : Constant  Value=123
  Chisel1 : Constant  Value=7.3
  Chisel2 : Constant  Value=0
  Constant A : MultiPortSwitch  SaturateOnIntegerOverflow=on  InputSameDT=on
  Constant B : MultiPortSwitch  SaturateOnIntegerOverflow=on  InputSameDT=on
  Constant C : MultiPortSwitch  SaturateOnIntegerOverflow=on  InputSameDT=on
  Cultivator : Constant  Value=32
  Cultivator1 : Constant  Value=1.9
  Cultivator2 : Constant  Value=0
  "Draft [N] " : Fcn  Expr=u[1]*(u[3]+u[4]*u[2]+u[5]*u[2]^2)*u[6]*u[7]
  Gain : Gain  Gain=.5
  Gain1 : Gain  Gain=.5
  Gain2 : Gain  Gain=.1
  Gain3 : Gain  Gain=.25
  MinMax : MinMax  Inputs=2
  MinMax1 : MinMax  Inputs=2
  Mux1 : Mux  Inputs=7
  Mux2 : Mux  Inputs=5
  Mux3 : Mux
  Mux5 : Mux
  No Hx2 Force : Constant  Value=0
  No Vy Force : Constant  Value=0
  Plow : Constant  Value=652
  Plow1 : Constant  Value=0
  Plow2 : Constant  Value=5.1
  Saturation : Saturate  UpperLimit=inf  LowerLimit=0
  Scope{,1..3} (4 alike) : Scope
      Scope settings: SaveName=ScopeData53
      Scope2 settings: YMin=0  YMax=3000
      Scope3 settings: SaveName=ScopeData2
  Sum1 : Sum  Inputs=-+  SaturateOnIntegerOverflow=on  OutDataTypeStr=Inherit: Same as first input
  Sum2 : Sum  Inputs=-+  SaturateOnIntegerOverflow=on  InputSameDT=on  OutDataTypeStr=Inherit: Same as first input
  Sum3 : Sum  Inputs=-+  SaturateOnIntegerOverflow=on  InputSameDT=on  OutDataTypeStr=Inherit: Same as first input
  Torque [N cm] : Fcn  Expr=(u(1)*u(2)+u(3)*u(4))/47.3075
  Vertical Force [N] : Fcn  Expr=(u(1)*u(2)+u(3)*u(4)+u(5)*u(2)*u(4))*10
  Width : MultiPortSwitch  SaturateOnIntegerOverflow=on  InputSameDT=on
  "Y1  " : MultiPortSwitch  SaturateOnIntegerOverflow=on  InputSameDT=on
  Y2 : MultiPortSwitch  SaturateOnIntegerOverflow=on  InputSameDT=on
  cm : Gain  Gain=100
  Vertical Force- BottomLink/Hitch (N) : Outport
  Horizontal Force- TopLink (N) : Outport  Port=2
  Horizontal Force- BottomLink/Hitch (N) : Outport  Port=3
  Total Horizontal Draft (N) : Outport  Port=4
  Vertical Position- BottomLink/Hitch (m) : Outport  Port=5
  Vertical Position- Top Link (m) : Outport  Port=6
  wires:
  1 - Sand/1 -> 3/2
  2 - Loam/1 -> 3/3
  3 - Clay/1 -> 3/4
  Chisel/1 -> Constant A/2
  Width (m) (Moldboard Plough)/1 -> Width/3
  Implement 1 Chisel Plough 2 Moldboard Plow 3 Field Cultivator/1 -> "Y1  "/1, Y2/1, Constant A/1, Constant B/1, Constant C/1, Width/1, 2/1, 1/1
  Speed (km/h)/1 -> Mux3/4, Mux2/4, Mux1/2
  C5 Vert/1 -> Mux2/5
  C3 Vert/1 -> Mux2/3
  C1 Vert/1 -> Mux2/1
  Mux2/1 -> Vertical Force [N]/1
  C1 Torque/1 -> Mux3/1
  C3 Torque/1 -> Mux3/3
  Mux3/1 -> Torque [N cm]/1
  3/1 -> Mux1/1
  Constant A/1 -> Mux1/3
  Constant B/1 -> Mux1/4
  Constant C/1 -> Mux1/5
  Width/1 -> Mux1/6
  Mux1/1 -> "Draft [N] "/1
  "Draft [N] "/1 -> Saturation/1
  1/1 -> Gain/1
  2/1 -> Gain1/1
  No Vy Force/1 -> 1/2
  Vertical Force [N]/1 -> 1/3, 1/4
  No Hx2 Force/1 -> 2/2, 2/3
  Torque [N cm]/1 -> 2/4
  Sum1/1 -> Mux5/2, Horizontal Force- BottomLink/Hitch (N)/1
  Mux5/1 -> Scope1/1
  Sum2/1 -> "Y1  "/3, "Y1  "/4
  Depth (m)/1 -> Mux2/2, Mux3/2, cm/1, Scope3/1, Sum2/1, Sum3/1, Scope2/1
  Soil Type 1 Sand 2 Loam 3 Clay/1 -> 3/1
  Drawbar Height (m)/1 -> "Y1  "/2
  "Y1  "/1 -> Vertical Position- BottomLink/Hitch (m)/1
  Height Bottom Link (m) (at zero depth)/1 -> Sum2/2
  Y2/1 -> Vertical Position- Top Link (m)/1
  Top Link position (m)/1 -> Sum3/2
  Number Shanks (Chisel Plough)/1 -> Width/2
  Number Tine (Field Cultuvator)/1 -> Width/4
  Cultivator/1 -> Constant A/4
  Plow/1 -> Constant A/3
  Chisel2/1 -> Constant C/2
  Cultivator2/1 -> Constant C/4
  Plow2/1 -> Constant C/3
  Chisel1/1 -> Constant B/2
  Plow1/1 -> Constant B/3
  Cultivator1/1 -> Constant B/4
  Gain/1 -> Abs/1
  Sum3/1 -> Y2/4
  1 - Sand1/1 -> Y2/2, Y2/3
  cm/1 -> Mux1/7
  Gain1/1 -> Abs1/1
  Abs/1 -> MinMax/1
  Abs1/1 -> MinMax1/1
  Gain2/1 -> MinMax/2
  Gain3/1 -> MinMax1/2
  MinMax/1 -> Mux5/1, Vertical Force- BottomLink/Hitch (N)/1
  MinMax1/1 -> Horizontal Force- TopLink (N)/1, Mux5/3
  Saturation/1 -> Scope/1, Sum1/2, Mux5/4, Total Horizontal Draft (N)/1, Gain2/1, Gain3/1
